simulink model "observer123"  (R2015b)
settings: Solver=ode45  StartTime=0.0  StopTime=10.0  RelTol=1e-3
values from neighbouring files (symbols this model uses):
  A = [-1 -1 0;-1 0 0;0 -1 -1]    [FULLORDERUNKNOWN.m]    (also in OBSERVER.m = [0 20.6;1 0]; functional.m = [-10 2 0 1 0; 1 -1 0 0 1;1 0 -5 3 4; -3 1 1 -8 3; -2 -4 0 2 ; lmi.m = [-10 2 0 1 0; 1 -1 0 0 1;1 0 -5 3 4; -3 1 1 -8 3; -2 -4 0 2 ; reduced_observer.m = [1 0 -2 2 0 0 -8 -6 -2;0 -1 3 18 41 -10 -19 -28 4; 1 2 3 4 4)
  B = [1;2;3]    [FULLORDERUNKNOWN.m]    (also in OBSERVER.m = [0;1]; functional.m = [1;2;3;4;5]; lmi.m = [1;2;3;4;5]; reduced_observer.m = [1;2;3;4;5;6;7;8;9])
  C = [1 0 0;0 0 1]    [FULLORDERUNKNOWN.m]    (also in OBSERVER.m = [0 1]; functional.m = [1 0 0 0 0;0 1 0 0 0]; lmi.m = [1 0 0 0 0;0 1 0 0 0]; reduced_observer.m = [1 0 0 0 0 0 0 0 0;0 1 0 0 0 0 0 0 0; 0 0 1 0 0 0 0 0 0])
  k = place(A,B,e)    [FULLORDERUNKNOWN.m]    (also in OBSERVER.m; functional.m = cell(Y,1); reduced_observer.m)
  L = L'    [FULLORDERUNKNOWN.m]    (also in OBSERVER.m = l'; reduced_observer.m)
settings Model: Creator=MAYANK  LastModifiedBy=deepika
settings DataIOCC: SaveFormat=Array
settings HardwareCC: ProdBitPerPointer=32  ProdLargestAtomicFloat=None  ProdIntDivRoundTo=Undefined  ProdEndianess=Unspecified  ProdWordSize=32  ProdHWDeviceType=32-bit Generic
settings GRTTargetCC: GeneratePreprocessorConditionals=Disable all
settings ConfigComp: CovModelRefEnable=Off

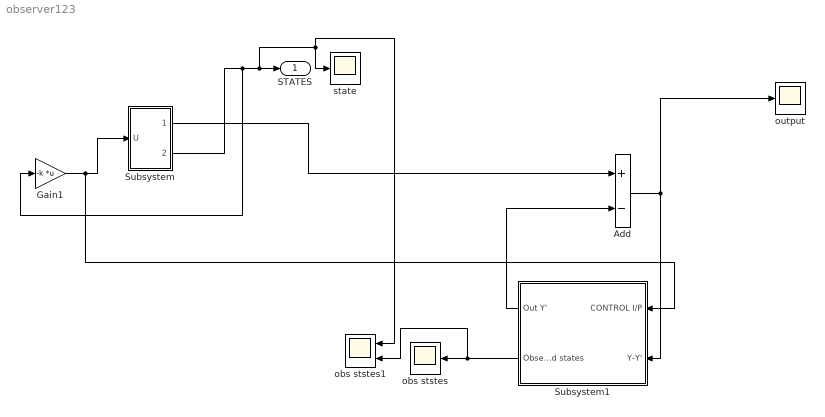
== system observer123 ==
  Add : Sum  Inputs=+-
  Gain1 : Gain  Gain=-k  Multiplication=Matrix(K*u)
  Subsystem : Subsystem
  Subsystem1 : Subsystem
  obs ststes : Scope
  obs ststes1 : Scope  NumInputPorts=2
  output : Scope
  state : Scope
  STATES : Outport
  wires:
  Subsystem/1(OUTPUT) -> Add/1
  Subsystem1/1(Out Y') -> Add/2
  Add/1 -> Subsystem1/2(Y-Y'), output/1
  Gain1/1 -> Subsystem1/1(CONTROL I/P), Subsystem/1(U)
  Subsystem1/2(Observed states) -> obs ststes1/2, obs ststes/1
  Subsystem/2(STATES) -> Gain1/1, state/1, obs ststes1/1, STATES/1

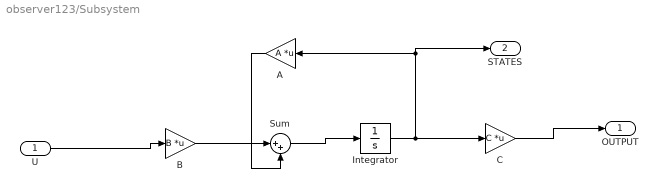
== system observer123/Subsystem ==
  U : Inport
  A : Gain  Gain=A  Multiplication=Matrix(K*u)
  B : Gain  Gain=B  Multiplication=Matrix(K*u)
  C : Gain  Gain=C  Multiplication=Matrix(K*u)
  Integrator : Integrator  InitialCondition=[1;1]
  Sum : Sum  Inputs=|++
  OUTPUT : Outport
  STATES : Outport  Port=2
  wires:
  B/1 -> Sum/1
  U/1 -> B/1
  Sum/1 -> Integrator/1
  Integrator/1 -> C/1, STATES/1, A/1
  A/1 -> Sum/2
  C/1 -> OUTPUT/1

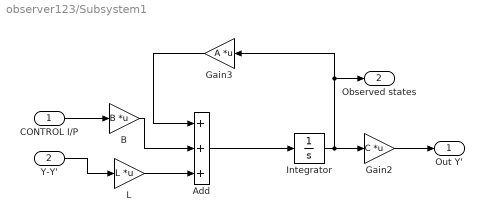
== system observer123/Subsystem1 ==
  CONTROL I/P : Inport
  Y-Y' : Inport  Port=2
  Add : Sum  Inputs=+++
  B : Gain  Gain=B  Multiplication=Matrix(K*u)
  Gain2 : Gain  Gain=C  Multiplication=Matrix(K*u)
  Gain3 : Gain  Gain=A  Multiplication=Matrix(K*u)
  Integrator : Integrator  InitialCondition=[1;1]
  L : Gain  Gain=L  Multiplication=Matrix(K*u)
  Out Y' : Outport
  Observed states : Outport  Port=2
  wires:
  B/1 -> Add/2
  CONTROL I/P/1 -> B/1
  Y-Y'/1 -> L/1
  Gain3/1 -> Add/1
  Gain2/1 -> Out Y'/1
  Integrator/1 -> Gain2/1, Observed states/1, Gain3/1
  Add/1 -> Integrator/1
  L/1 -> Add/3
